simulink library "DAEMOT_Lib"  (R2019b)
settings: Solver=ode45  StartTime=0.0  StopTime=10.0  FixedStep=0.1  RelTol=1e-3
undefined symbols (not defined in the file or in its folder): Controller, CP, Ctrl, Ctrl_Fcn, Elec1, f, F2, Fluid, lag1, Mission, Moody, PropellerProp, rev_comms_sink
libraries: $bdroot x200, instrumentlib x21, simulink x5, dspsigops x2
(part 9 of 13)

== system DAEMOT_Lib/Legacy Components/LabVIEW_UDP_old ==
  " " : Inport
  Bus Creator : BusCreator  Inputs=46
  Bus Selector : BusSelector  OutputSignals=Temp1_Enabled,Temp2_Enabled,Temp3_Enabled,Temp4_Enabled,Temp5_Enabled,Temp6_Enabled,Temp7_Enabled,Temp8_Enabled,Temp9_Enabled,Temp10_Enabled,Temp11_Enabled,Temp12_Enabled,Temp13_Enabled,Temp14_Enabled,Temp15_Enabled,Temp16_Enabled,FlowMeter1_Enabled,FlowMeter2_Enabled,FlowMeter3_Enabled,FlowMeter4_Enabled,FlowMeter5_Enabled,FlowMeter6_Enabled,FlowMeter7_Enabled,FlowMeter8_Enabled,Pump1,Pump2,Pump3,Pump4,Pump5,Pump6,Pump7,Pump8,Pump1_Enabled,Pump2_Enabled,Pump3_Enabled,Pump4_Enabled,Pump5_Enabled,Pump6_Enabled,Pump7_Enabled,Pump8_Enabled,Heater1,Heater2,Heater3,Heater4,Heater1_Enabled,Heater2_Enabled,Heater3_Enabled,Heater4_Enabled,Heater1_CM_Enabled,Heater2_CM_Enabled,Heater3_CM_Enabled,Heater4_CM_Enabled,Pressure1_Enabled,Pressure2_Enabled,Pressure3_Enabled,Pressure4_Enabled,Pressure5_Enabled,Pressure6_Enabled,Pressure7_Enabled,Chiller2,Chiller2_Enabled,Valve1_Enabled,Valve2_Enabled,Valve3_Enabled,Valve4_Enabled,Valve5_Enabled,Valve6_Enabled,Valve7_Enabled,Valve8_Enabled,Chiller1,Chiller1_Enabled  OutputAsBus=on
  Bus to Vector : BusToVector
  Demux : Demux  Outputs=46
  UDP Receive : instrumentlib/UDP Receive  Host=localhost  Port=61556  LocalPort=61557  EnablePortSharing=off  GetLatestData=off  DataSize=[48 1]  DataType=double  ASCIIFormatting=%f,  Terminator=LF  ByteOrder=BigEndian  EnableBlockingMode=on  Timeout=10  SampleTime=0.1  LocalAddress=0.0.0.0
      settings: SourceProductName=Instrument Control Toolbox
  UDP Send : instrumentlib/UDP Send  Host=localhost  Port=61556  LocalPort=61557  EnablePortSharing=off  ByteOrder=BigEndian  OutputDatagramPacketSize=512  EnableBlockingMode=on  LocalAddress=0.0.0.0
      settings: SourceProductName=Instrument Control Toolbox
  Zero-Order Hold : ZeroOrderHold  Commented=through  SampleTime=0.1
  Out : Outport  VectorParamsAs1DForOutWhenUnconnected=off
  wires:
  UDP Receive/1 -> Demux/1
  Demux/1 -> Bus Creator/1  "Temp1"
  Demux/2 -> Bus Creator/2  "Temp2"
  Bus Creator/1 -> Out/1
  Demux/3 -> Bus Creator/3  "Temp3"
  Demux/4 -> Bus Creator/4  "Temp4"
  Demux/5 -> Bus Creator/5  "Temp5"
  Demux/6 -> Bus Creator/6  "Temp6"
  Demux/7 -> Bus Creator/7  "Temp7"
  Demux/8 -> Bus Creator/8  "Temp8"
  Demux/9 -> Bus Creator/9  "Temp9"
  Demux/10 -> Bus Creator/10  "Temp10"
  Demux/11 -> Bus Creator/11  "Temp11"
  Demux/12 -> Bus Creator/12  "Temp12"
  Demux/13 -> Bus Creator/13  "Temp13"
  Demux/14 -> Bus Creator/14  "Temp14"
  Demux/15 -> Bus Creator/15  "Temp15"
  Demux/16 -> Bus Creator/16  "Temp16"
  Demux/17 -> Bus Creator/17  "FlowMeter1"
  Demux/18 -> Bus Creator/18  "FlowMeter2"
  Demux/19 -> Bus Creator/19  "FlowMeter3"
  Demux/20 -> Bus Creator/20  "FlowMeter4"
  Demux/21 -> Bus Creator/21  "FlowMeter5"
  Demux/22 -> Bus Creator/22  "FlowMeter6"
  Demux/23 -> Bus Creator/23  "FlowMeter7"
  Demux/24 -> Bus Creator/24  "FlowMeter8"
  Demux/25 -> Bus Creator/25  "Pump1"
  Demux/26 -> Bus Creator/26  "Pump2"
  Demux/27 -> Bus Creator/27  "Pump3"
  Demux/28 -> Bus Creator/28  "Pump4"
  Demux/29 -> Bus Creator/29  "Pump5"
  Demux/30 -> Bus Creator/30  "Pump6"
  Demux/31 -> Bus Creator/31  "Pump7"
  Demux/32 -> Bus Creator/32  "Pump8"
  Demux/33 -> Bus Creator/33  "Heater1"
  Demux/34 -> Bus Creator/34  "Heater2"
  Demux/35 -> Bus Creator/35  "Heater3"
  Demux/36 -> Bus Creator/36  "Heater4"
  Demux/37 -> Bus Creator/37  "Pressure1"
  Demux/38 -> Bus Creator/38  "Pressure2"
  " "/1 -> Bus Selector/1
  Zero-Order Hold/1 -> UDP Send/1
  Bus Selector/1 -> Bus to Vector/1
  Bus to Vector/1 -> Zero-Order Hold/1
  Demux/39 -> Bus Creator/39  "Pressure3"
  Demux/40 -> Bus Creator/40  "Pressure4"
  Demux/41 -> Bus Creator/41  "Pressure5"
  Demux/42 -> Bus Creator/42  "Pressure6"
  Demux/43 -> Bus Creator/43  "Pressure7"
  Demux/44 -> Bus Creator/44  "Chiller1_flow"
  Demux/45 -> Bus Creator/45  "Chiller1_temp"
  Demux/46 -> Bus Creator/46  "RunTime"

== system DAEMOT_Lib/Legacy Components/Load ==
  In1 : Inport
  In2 : Inport  Port=2
  Bus Selector : BusSelector  OutputSignals=V,I
  Constant : Constant  Value=0
  Constant1 : Constant  Value=0
  Data_Sink1 : $bdroot/Support Functions/Data_Sink
  Divide : Product  Inputs=/
  Gain : Gain  Gain=1000
  P : Constant  Value=P_max
  Product : Product
  Product1 : Product
  Sink1 : $bdroot/Support Functions/Sink
  Switch : Switch  Criteria=u2 > Threshold
  Switch1 : Switch  Criteria=u2 > Threshold
  Terminator3 : Terminator
  b1 : BusCreator  Inputs=1
  wires:
  Bus Selector/1 -> Switch1/2, Divide/1, Switch/2  "<V>"
  Bus Selector/2 -> Terminator3/1  "<I>"
  Product1/1 -> Gain/1  "I"
  In1/1 -> Bus Selector/1
  P/1 -> Product/1
  In2/1 -> Product/2
  Switch/1 -> Product1/1
  Divide/1 -> Switch/1
  Constant/1 -> Switch/3
  b1/1 -> Data_Sink1/1
  Switch1/1 -> b1/1, Product1/2  "Power"
  Constant1/1 -> Switch1/3
  Product/1 -> Switch1/1  "Power"
  Gain/1 -> Sink1/1

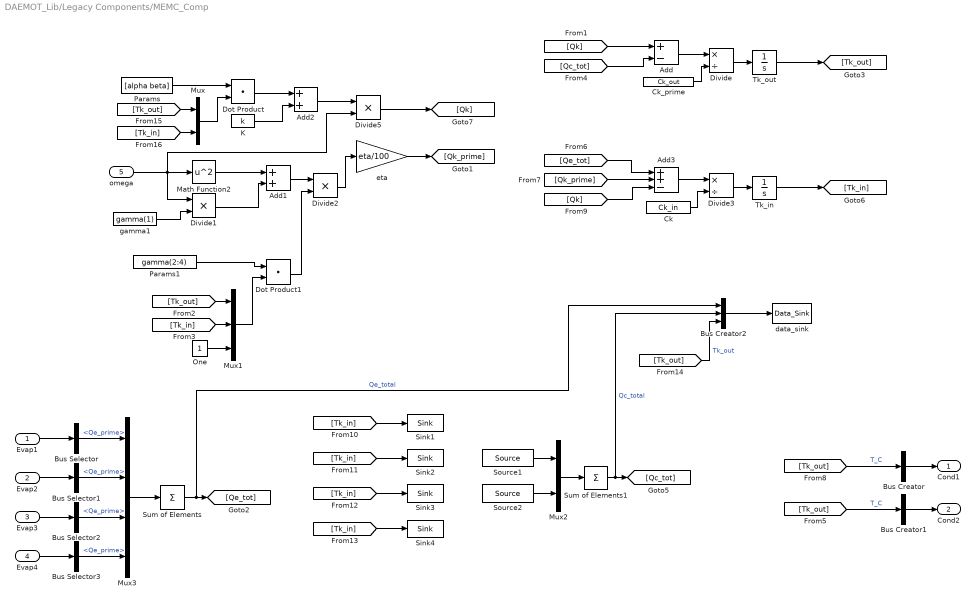
== system DAEMOT_Lib/Legacy Components/MEMC_Comp ==
  Evap1 : Inport
  Evap2 : Inport  Port=2
  Evap3 : Inport  Port=3
  Evap4 : Inport  Port=4
  omega : Inport  Port=5
  Add : Sum  Inputs=+-
  Add1 : Sum
  Add2 : Sum
  Add3 : Sum  Inputs=++-
  Bus Creator : BusCreator  Inputs=1
  Bus Creator1 : BusCreator  Inputs=1
  Bus Creator2 : BusCreator  Inputs=3
  Bus Selector{,1..3} (4 alike) : BusSelector  OutputSignals=Qe_prime
  Ck : Constant  Value=Ck_in
  Ck_prime : Constant  Value=Ck_out
  Divide : Product  Inputs=*/
  Divide1 : Product  Inputs=**
  Divide2 : Product  Inputs=**
  Divide3 : Product  Inputs=*/
  Divide5 : Product  Inputs=**
  Dot Product : DotProduct  InputSameDT=on  OutDataTypeStr=Inherit: Inherit via internal rule
  Dot Product1 : DotProduct  InputSameDT=on  OutDataTypeStr=Inherit: Inherit via internal rule
  K : Constant  Value=k
  Math Function2 : Math  Operator=square  SaturateOnIntegerOverflow=on
  Mux : Mux  Inputs=2
  Mux1 : Mux  Inputs=3
  Mux2 : Mux  Inputs=2
  Mux3 : Mux
  One : Constant
  Params : Constant  Value=[alpha beta]
  Params1 : Constant  Value=gamma(2:4)
  Sink{1..4} (4 alike) : $bdroot/Support Functions/Sink
  Source1 : $bdroot/Support Functions/Source
  Source2 : $bdroot/Support Functions/Source
  Sum of Elements : Sum  Inputs=+
  Sum of Elements1 : Sum  Inputs=+
  Tk_in : Integrator  InitialCondition=Tk_in_init
  Tk_out : Integrator  InitialCondition=Tk_out_init
  data_sink : $bdroot/Support Functions/Data_Sink
  eta : Gain  Gain=eta/100
  gamma1 : Constant  Value=gamma(1)
  Cond1 : Outport  VectorParamsAs1DForOutWhenUnconnected=off
  Cond2 : Outport  Port=2  VectorParamsAs1DForOutWhenUnconnected=off
  wires:
  [Tk_in] -> Sink4/1
  [Tk_in] -> Sink3/1
  [Tk_in] -> Sink2/1
  [Tk_in] -> Sink1/1
  [Qk] -> Add3/3
  Tk_in/1 -> [Tk_in]
  Add3/1 -> Divide3/1
  [Qk_prime] -> Add3/2
  [Qe_tot] -> Add3/1
  Divide3/1 -> Tk_in/1
  Ck/1 -> Divide3/2
  Sum of Elements1/1 -> Bus Creator2/2, [Qc_tot]  "Qc_total"
  Mux2/1 -> Sum of Elements1/1
  Source2/1 -> Mux2/2
  Source1/1 -> Mux2/1
  [Tk_out] -> Bus Creator1/1  "T_C"
  Bus Creator1/1 -> Cond2/1
  [Tk_out] -> Bus Creator/1  "T_C"
  Bus Creator/1 -> Cond1/1
  Tk_out/1 -> [Tk_out]
  Add/1 -> Divide/1
  [Qc_tot] -> Add/2
  [Qk] -> Add/1
  Divide/1 -> Tk_out/1
  Ck_prime/1 -> Divide/2
  Mux/1 -> Dot Product/2
  Params/1 -> Dot Product/1
  [Tk_in] -> Mux/2
  [Tk_out] -> Mux/1
  Divide5/1 -> [Qk]
  eta/1 -> [Qk_prime]
  Divide2/1 -> eta/1
  omega/1 -> Math Function2/1, Divide1/1, Divide5/2
  Add1/1 -> Divide2/1
  Math Function2/1 -> Add1/1
  Divide1/1 -> Add1/2
  gamma1/1 -> Divide1/2
  Mux1/1 -> Dot Product1/2
  Params1/1 -> Dot Product1/1
  [Tk_in] -> Mux1/2
  [Tk_out] -> Mux1/1
  Dot Product1/1 -> Divide2/2
  Dot Product/1 -> Add2/1
  K/1 -> Add2/2
  Add2/1 -> Divide5/1
  One/1 -> Mux1/3
  Sum of Elements/1 -> Bus Creator2/1, [Qe_tot]  "Qe_total"
  Mux3/1 -> Sum of Elements/1
  Bus Selector/1 -> Mux3/1  "<Qe_prime>"
  Bus Selector3/1 -> Mux3/4  "<Qe_prime>"
  Bus Selector1/1 -> Mux3/2  "<Qe_prime>"
  Bus Selector2/1 -> Mux3/3  "<Qe_prime>"
  Evap2/1 -> Bus Selector1/1
  Evap3/1 -> Bus Selector2/1
  Evap4/1 -> Bus Selector3/1
  Evap1/1 -> Bus Selector/1
  Bus Creator2/1 -> data_sink/1
  [Tk_out] -> Bus Creator2/3  "Tk_out"

== system DAEMOT_Lib/Legacy Components/MEMC_Valves ==
  Cond2 : Inport
  Cond1 : Inport  Port=2
  Add : Sum  Inputs=+-
  Bus Creator{,1..4} (5 alike) : BusCreator  Inputs=1
  Bus Selector1 : BusSelector  OutputSignals=Qc_prime
  Bus Selector2 : BusSelector  OutputSignals=Qc_prime
  Cv : Constant  Value=Cv
  Divide : Product  Inputs=*/
  Mux1 : Mux
  Mux2 : Mux  Inputs=2
  Sink1 : $bdroot/Support Functions/Sink
  Sink2 : $bdroot/Support Functions/Sink
  Source{1..4} (4 alike) : $bdroot/Support Functions/Source
  Sum of Elements1 : Sum  Inputs=+
  Sum of Elements4 : Sum  Inputs=+
  Tv : Integrator  InitialCondition=T_init
  data_sink : $bdroot/Support Functions/Data_Sink
  Evap4 : Outport  VectorParamsAs1DForOutWhenUnconnected=off
  Evap3 : Outport  Port=2  VectorParamsAs1DForOutWhenUnconnected=off
  Evap2 : Outport  Port=3  VectorParamsAs1DForOutWhenUnconnected=off
  Evap1 : Outport  Port=4  VectorParamsAs1DForOutWhenUnconnected=off
  wires:
  Tv/1 -> Bus Creator4/1, [Tv]  "Temp_C"
  Add/1 -> Divide/1
  [Qe_tot] -> Add/2
  [Qc_prime_tot] -> Add/1
  Divide/1 -> Tv/1
  Cv/1 -> Divide/2
  [Tv] -> Bus Creator/1, Bus Creator1/1, Bus Creator2/1, Bus Creator3/1  "T_C"
  Mux1/1 -> Sum of Elements4/1
  Sum of Elements4/1 -> [Qe_tot]
  Source4/1 -> Mux1/4
  Source3/1 -> Mux1/3
  Source1/1 -> Mux1/1
  Source2/1 -> Mux1/2
  Sum of Elements1/1 -> [Qc_prime_tot]
  Mux2/1 -> Sum of Elements1/1
  Bus Selector2/1 -> Mux2/2  "<Qc_prime>"
  Bus Selector1/1 -> Mux2/1  "<Qc_prime>"
  Cond2/1 -> Bus Selector1/1
  [Tv] -> Sink2/1, Sink1/1
  Bus Creator/1 -> Evap4/1
  Cond1/1 -> Bus Selector2/1
  Bus Creator1/1 -> Evap3/1
  Bus Creator2/1 -> Evap2/1
  Bus Creator3/1 -> Evap1/1
  Bus Creator4/1 -> data_sink/1

== system DAEMOT_Lib/Legacy Components/Pipe_M_to_M ==
  In1 : Inport
  In2 : Inport  Port=2
  Add1 : Sum
  Add5 : Sum
  Bus Creator2 : BusCreator  Inputs=3
  Constant : Constant  Value=4/(pi*D)
  Constant1 : Constant  Value=e/D
  Display : Display
  Display1 : Display
  Display2 : Display
  Divide5 : Product  Inputs=**/
  From1 : From  Commented=on  GotoTag=T_out
      settings: CloseFcn=tagdialog Close
  Gain1 : Gain  Gain=1/Fluid.Bulk_Mod
  Gain2 : Gain  Gain=0.5
  Gain3 : Gain  Gain=0.5
  Integrate1 : Integrator  InitialCondition=P_init
  Memory1 : Memory  Commented=on  InitialCondition=[Tout_init]
  Pipe_M_to_M : MATLAB Function  TreatAsAtomicUnit=on
  Props : Subsystem
  Sink1 : $bdroot/Support Functions/Sink
  Source1 : $bdroot/Support Functions/Source
  Terminator : Terminator
  Terminator1 : Terminator
  Terminator2 : Terminator
  b1 : BusCreator  Inputs=3
  data_sink1 : $bdroot/Support Functions/Data_Sink
  gb1 : BusSelector  OutputSignals=mdot_kgps,T_C,P_kPa
  n-D Lookup Table5 : Lookup_n-D  BreakpointsForDimension1=Moody.Re_vec  BreakpointsForDimension2=Moody.eD_vec  BreakpointsForDimension3=[5, 7]  Table=Moody.f  ExtrapMethod=Clip  UseLastTableValue=on  RndMeth=Simplest  InputSameDT=on
  n-D Lookup Table9 : Lookup_n-D  BreakpointsForDimension1=Fluid.P  BreakpointsForDimension2=Fluid.T  BreakpointsForDimension3=[5, 7]  Table=Fluid.Mu_pt  RndMeth=Simplest  InputSameDT=on
  Out1 : Outport  VectorParamsAs1DForOutWhenUnconnected=off
  wires:
  b1/1 -> Out1/1
  [Mdot_out] -> b1/1  "mdot_kgps"
  gb1/2 -> [T_in]  "<T_C>"
  [T_out] -> b1/2  "T_C"
  gb1/1 -> [Mdot_in]  "<mdot_kgps>"
  In1/1 -> gb1/1
  [P_out] -> b1/3  "P_kPa"
  gb1/3 -> Terminator/1  "<P_kPa>"
  [P_in] -> Sink1/1
  Source1/1 -> [Mdot_out]
  In2/1 -> [T_amb]
  Bus Creator2/1 -> data_sink1/1
  [T_out] -> Bus Creator2/1  "T_out"
  [P_in] -> Bus Creator2/2  "P_in"
  [T_amb] -> Terminator1/1
  [T_in] -> [T_out]
  [Mdot_in] -> Add5/1, Pipe_M_to_M/2(Mdot_in)
  [Mdot_out] -> Add5/2, Pipe_M_to_M/3(Mdot_out)
  [T_in] -> Add1/2, Add1/1
  From1/1 -> Memory1/1
  Add1/1 -> Gain2/1
  Gain2/1 -> n-D Lookup Table9/2, Props/2(T)
  [P] -> Props/1(P), n-D Lookup Table9/1
  Add5/1 -> Gain3/1
  Constant/1 -> Divide5/1
  Gain3/1 -> Divide5/2
  Divide5/1 -> Display/1, n-D Lookup Table5/1  "Re"
  Constant1/1 -> Display2/1, n-D Lookup Table5/2
  n-D Lookup Table5/1 -> Pipe_M_to_M/6(f), Display1/1
  Props/1(Rho) -> Gain1/1, Pipe_M_to_M/4(Rho)
  Integrate1/1 -> [P], Pipe_M_to_M/1(x)
  Pipe_M_to_M/1(x_dot) -> Integrate1/1
  [P_out] -> Bus Creator2/3  "P_out"
  Pipe_M_to_M/2(P_in) -> [P_in]
  Pipe_M_to_M/3(P_out) -> [P_out]
  n-D Lookup Table9/1 -> Divide5/3  "mu"
  Gain1/1 -> Pipe_M_to_M/5(dRho_dP)
  Props/2(dRho_dP) -> Terminator2/1

== system DAEMOT_Lib/Legacy Components/Pipe_M_to_P ==
  In1 : Inport
  In2 : Inport  Port=2
  Add1 : Sum
  Bus Creator2 : BusCreator  Inputs=3
  Constant : Constant  Value=4/(pi*D)
  Constant1 : Constant  Value=e/D
  Display : Display
  Display1 : Display
  Display2 : Display
  Divide5 : Product  Inputs=**/
  From1 : From  Commented=on  GotoTag=T_out
      settings: CloseFcn=tagdialog Close
  Gain1 : Gain  Gain=1/Fluid.Bulk_Mod
  Gain2 : Gain  Gain=0.5
  Integrate : Integrator  InitialCondition=P_init
  Memory1 : Memory  Commented=on  InitialCondition=[Tout_init]
  Pipe_P_to_M : MATLAB Function  TreatAsAtomicUnit=on
  Sink1 : $bdroot/Support Functions/Sink
  Source1 : $bdroot/Support Functions/Source
  Terminator1 : Terminator
  Terminator2 : Terminator
  b2 : BusCreator  Inputs=3
  data_sink1 : $bdroot/Support Functions/Data_Sink
  gb2 : BusSelector  OutputSignals=mdot_kgps,T_C,P_kPa
  n-D Lookup Table2 : Lookup_n-D  BreakpointsForDimension1=Fluid.P  BreakpointsForDimension2=Fluid.T  BreakpointsForDimension3=[5, 7]  Table=Fluid.Rho_pt  ExtrapMethod=Clip  UseLastTableValue=on  RndMeth=Simplest  InputSameDT=on
  n-D Lookup Table5 : Lookup_n-D  BreakpointsForDimension1=Moody.Re_vec  BreakpointsForDimension2=Moody.eD_vec  BreakpointsForDimension3=[5, 7]  Table=Moody.f  ExtrapMethod=Clip  UseLastTableValue=on  RndMeth=Simplest  InputSameDT=on
  n-D Lookup Table9 : Lookup_n-D  BreakpointsForDimension1=Fluid.P  BreakpointsForDimension2=Fluid.T  BreakpointsForDimension3=[5, 7]  Table=Fluid.Mu_pt  RndMeth=Simplest  InputSameDT=on
  Out1 : Outport  VectorParamsAs1DForOutWhenUnconnected=off
  wires:
  Bus Creator2/1 -> data_sink1/1
  [T_out] -> Bus Creator2/1  "T_out"
  [T_amb] -> Terminator1/1
  [T_in] -> [T_out]
  From1/1 -> Memory1/1
  Add1/1 -> Gain2/1
  Gain2/1 -> n-D Lookup Table2/2, n-D Lookup Table9/2
  [P_in] -> n-D Lookup Table2/1, n-D Lookup Table9/1
  Constant/1 -> Divide5/1
  Divide5/1 -> Display/1, n-D Lookup Table5/1  "Re"
  Constant1/1 -> Display2/1, n-D Lookup Table5/2
  n-D Lookup Table5/1 -> Pipe_P_to_M/6(f), Display1/1
  n-D Lookup Table2/1 -> Pipe_P_to_M/4(Rho), Gain1/1
  [T_in] -> Add1/2, Add1/1
  n-D Lookup Table9/1 -> Divide5/3  "mu"
  [Mdot] -> Bus Creator2/2  "Mdot"
  Pipe_P_to_M/2(Mdot) -> [Mdot]
  [P_in] -> Bus Creator2/3  "P_out"
  [Mdot_up] -> Divide5/2
  Pipe_P_to_M/1(x_dot) -> Integrate/1
  Integrate/1 -> Pipe_P_to_M/1(x), [P_in]
  b2/1 -> Out1/1
  [Mdot] -> b2/1  "mdot_kgps"
  gb2/2 -> [T_in]  "<T_C>"
  [T_out] -> b2/2  "T_C"
  gb2/1 -> [Mdot_up]  "<mdot_kgps>"
  In1/1 -> gb2/1
  [P_out] -> b2/3  "P_kPa"
  gb2/3 -> Terminator2/1  "<P_kPa>"
  [P_in] -> Sink1/1
  Source1/1 -> [P_out]
  In2/1 -> [T_amb]
  [P_out] -> Pipe_P_to_M/2(P_out)
  [Mdot_up] -> Pipe_P_to_M/3(Mdot_up)
  Gain1/1 -> Pipe_P_to_M/5(dRho_dP)

== system DAEMOT_Lib/Legacy Components/Pipe_P_to_M1 ==
  In1 : Inport
  Bus Creator2 : BusCreator  Inputs=3
  Constant2 : Constant  Value=Fluid.Bulk_Mod
  Demux : Demux  Outputs=2
  Integrate : Integrator  InitialCondition=[T_init P_init]
  Mdot : MATLAB Function  TreatAsAtomicUnit=on
  Pipe_P_to_M : MATLAB Function  TreatAsAtomicUnit=on
  Sink1 : $bdroot/Support Functions/Sink
  Source1 : $bdroot/Support Functions/Source
  Terminator3 : Terminator
  b2 : BusCreator  Inputs=3
  data_sink1 : $bdroot/Support Functions/Data_Sink
  gb2 : BusSelector  OutputSignals=mdot_kgps,T_C,P_kPa
  n-D Lookup Table2 : Lookup_n-D  BreakpointsForDimension1=Fluid.P  BreakpointsForDimension2=Fluid.T  BreakpointsForDimension3=[5, 7]  Table=Fluid.Rho_pt  ExtrapMethod=Clip  UseLastTableValue=on  RndMeth=Simplest  InputSameDT=on
  Out1 : Outport  VectorParamsAs1DForOutWhenUnconnected=off
  wires:
  Bus Creator2/1 -> data_sink1/1
  [T_out] -> Bus Creator2/1  "T_out"
  [T_out] -> n-D Lookup Table2/2
  [P_out] -> n-D Lookup Table2/1
  n-D Lookup Table2/1 -> Pipe_P_to_M/5(Rho), Mdot/3(Rho)
  [Mdot] -> Bus Creator2/2  "Mdot"
  [P_out] -> Bus Creator2/3  "P_out"
  Pipe_P_to_M/1(x_dot) -> Integrate/1
  Integrate/1 -> Pipe_P_to_M/1(x), Demux/1
  b2/1 -> Out1/1
  [Mdot_down] -> b2/1  "mdot_kgps"
  gb2/2 -> [T_in]  "<T_C>"
  [T_out] -> b2/2  "T_C"
  gb2/1 -> Terminator3/1  "<mdot_kgps>"
  In1/1 -> gb2/1
  [P_out] -> b2/3  "P_kPa"
  gb2/3 -> [P_in]  "<P_kPa>"
  [Mdot] -> Sink1/1
  Source1/1 -> [Mdot_down]
  [Mdot_down] -> Pipe_P_to_M/3(Mdot_down)
  Constant2/1 -> Pipe_P_to_M/6(E_fluid)
  [T_in] -> Pipe_P_to_M/2(T_in)
  [P_in] -> Mdot/1(P_in)
  [P_out] -> Mdot/2(P_out)
  Mdot/1(Mdot) -> Pipe_P_to_M/4(Mdot), [Mdot]
  Demux/2 -> [P_out]
  Demux/1 -> [T_out]

== system DAEMOT_Lib/Legacy Components/Pipe_P_to_M_Wall ==
  In1 : Inport
  In2 : Inport  Port=2
  Bus Creator2 : BusCreator  Inputs=4
  Constant2 : Constant  Value=Fluid.Bulk_Mod
  Demux : Demux  Outputs=2
  Integrate : Integrator  InitialCondition=[T_init P_init]
  Mdot : MATLAB Function  TreatAsAtomicUnit=on
  Pipe_P_to_M : MATLAB Function  TreatAsAtomicUnit=on
  Sink1 : $bdroot/Support Functions/Sink
  Sink2 : $bdroot/Support Functions/Sink
  Source1 : $bdroot/Support Functions/Source
  Terminator3 : Terminator
  b2 : BusCreator  Inputs=3
  bus : BusSelector  OutputSignals=T_wall
  data_sink1 : $bdroot/Support Functions/Data_Sink
  gb2 : BusSelector  OutputSignals=mdot_kgps,T_C,P_kPa
  n-D Lookup Table1 : Lookup_n-D  BreakpointsForDimension1=Fluid.P  BreakpointsForDimension2=Fluid.T  BreakpointsForDimension3=[5, 7]  Table=Fluid.C_pt  ExtrapMethod=Clip  UseLastTableValue=on  RndMeth=Simplest  InputSameDT=on
  n-D Lookup Table2 : Lookup_n-D  BreakpointsForDimension1=Fluid.P  BreakpointsForDimension2=Fluid.T  BreakpointsForDimension3=[5, 7]  Table=Fluid.Rho_pt  ExtrapMethod=Clip  UseLastTableValue=on  RndMeth=Simplest  InputSameDT=on
  n-D Lookup Table8 : Lookup_n-D  BreakpointsForDimension1=Fluid.P  BreakpointsForDimension2=Fluid.T  BreakpointsForDimension3=[5, 7]  Table=Fluid.K_pt  ExtrapMethod=Clip  UseLastTableValue=on  RndMeth=Simplest  InputSameDT=on
  n-D Lookup Table9 : Lookup_n-D  BreakpointsForDimension1=Fluid.P  BreakpointsForDimension2=Fluid.T  BreakpointsForDimension3=[5, 7]  Table=Fluid.Mu_pt  ExtrapMethod=Clip  UseLastTableValue=on  RndMeth=Simplest  InputSameDT=on
  Out1 : Outport  VectorParamsAs1DForOutWhenUnconnected=off
  wires:
  Bus Creator2/1 -> data_sink1/1
  [T_out] -> Bus Creator2/1  "T_out"
  In2/1 -> bus/1
  [T_out] -> n-D Lookup Table1/2, n-D Lookup Table8/2, n-D Lookup Table9/2, n-D Lookup Table2/2
  n-D Lookup Table2/1 -> Pipe_P_to_M/9(Rho), Mdot/3(Rho)
  [Mdot] -> Bus Creator2/2  "Mdot"
  [P_out] -> Bus Creator2/3  "P_out"
  Pipe_P_to_M/1(x_dot) -> Integrate/1
  Integrate/1 -> Pipe_P_to_M/1(x), Demux/1
  b2/1 -> Out1/1
  [Mdot_down] -> b2/1  "mdot_kgps"
  gb2/2 -> [T_in]  "<T_C>"
  [T_out] -> b2/2  "T_C"
  gb2/1 -> Terminator3/1  "<mdot_kgps>"
  In1/1 -> gb2/1
  [P_out] -> b2/3  "P_kPa"
  gb2/3 -> [P_in]  "<P_kPa>"
  [Mdot] -> Sink1/1
  Source1/1 -> [Mdot_down]
  [Mdot_down] -> Pipe_P_to_M/3(Mdot_down)
  Constant2/1 -> Pipe_P_to_M/5(E_fluid)
  [T_in] -> Pipe_P_to_M/2(T_in)
  [P_in] -> Mdot/1(P_in)
  [P_out] -> Mdot/2(P_out)
  Mdot/1(Mdot) -> Pipe_P_to_M/4(Mdot), [Mdot]
  Demux/2 -> [P_out]
  Demux/1 -> [T_out]
  n-D Lookup Table9/1 -> Pipe_P_to_M/6(mu)
  n-D Lookup Table1/1 -> Pipe_P_to_M/8(Cp)
  n-D Lookup Table8/1 -> Pipe_P_to_M/7(k)
  [P_out] -> n-D Lookup Table2/1, n-D Lookup Table1/1, n-D Lookup Table9/1, n-D Lookup Table8/1
  Pipe_P_to_M/2(Q_kW) -> [Q_fluid]
  [Q_fluid] -> Bus Creator2/4  "Q"
  [Q_fluid] -> Sink2/1
  bus/1 -> Pipe_P_to_M/10(T_wall)  "<T_wall>"

== system DAEMOT_Lib/Legacy Components/Pipe_P_to_M_with_Heat_Load ==
  In1 : Inport
  Q : Inport  Port=2
  Bus Creator2 : BusCreator  Inputs=4
  Bus Selector : BusSelector  OutputSignals=Q_kW,Temp
  Constant2 : Constant  Value=Fluid.Bulk_Mod
  Demux : Demux  Outputs=2
  Integrate : Integrator  InitialCondition=[T_init P_init]
  Mdot : MATLAB Function  TreatAsAtomicUnit=on
  Pipe_P_to_M : MATLAB Function  TreatAsAtomicUnit=on
  Sink1 : $bdroot/Support Functions/Sink
  Sink2 : $bdroot/Support Functions/Sink
  Source1 : $bdroot/Support Functions/Source
  Terminator : Terminator
  Terminator3 : Terminator
  b2 : BusCreator  Inputs=3
  data_sink1 : $bdroot/Support Functions/Data_Sink
  gb2 : BusSelector  OutputSignals=mdot_kgps,T_C,P_kPa
  n-D Lookup Table1 : Lookup_n-D  BreakpointsForDimension1=Fluid.P  BreakpointsForDimension2=Fluid.T  BreakpointsForDimension3=[5, 7]  Table=Fluid.C_pt  ExtrapMethod=Clip  UseLastTableValue=on  RndMeth=Simplest  InputSameDT=on
  n-D Lookup Table2 : Lookup_n-D  BreakpointsForDimension1=Fluid.P  BreakpointsForDimension2=Fluid.T  BreakpointsForDimension3=[5, 7]  Table=Fluid.Rho_pt  ExtrapMethod=Clip  UseLastTableValue=on  RndMeth=Simplest  InputSameDT=on
  Out1 : Outport  VectorParamsAs1DForOutWhenUnconnected=off
  wires:
  [Q_Load] -> Pipe_P_to_M/7(Q_load)
  [T_out] -> Sink2/1
  Bus Selector/2 -> Terminator/1  "<Temp>"
  Q/1 -> Bus Selector/1
  Bus Selector/1 -> [Q_Load]  "<Q_kW>"
  Bus Creator2/1 -> data_sink1/1
  [T_out] -> Bus Creator2/1  "T_out"
  [T_out] -> n-D Lookup Table1/2, n-D Lookup Table2/2
  [P_out] -> n-D Lookup Table1/1, n-D Lookup Table2/1
  n-D Lookup Table2/1 -> Pipe_P_to_M/5(Rho), Mdot/3(Rho)
  [Mdot] -> Bus Creator2/2  "Mdot"
  [P_out] -> Bus Creator2/3  "P_out"
  Pipe_P_to_M/1(x_dot) -> Integrate/1
  Integrate/1 -> Pipe_P_to_M/1(x), Demux/1
  b2/1 -> Out1/1
  [Mdot_down] -> b2/1  "mdot_kgps"
  gb2/2 -> [T_in]  "<T_C>"
  [T_out] -> b2/2  "T_C"
  gb2/1 -> Terminator3/1  "<mdot_kgps>"
  In1/1 -> gb2/1
  [P_out] -> b2/3  "P_kPa"
  gb2/3 -> [P_in]  "<P_kPa>"
  [Mdot] -> Sink1/1
  Source1/1 -> [Mdot_down]
  [Mdot_down] -> Pipe_P_to_M/3(Mdot_down)
  Constant2/1 -> Pipe_P_to_M/6(E_fluid)
  [T_in] -> Pipe_P_to_M/2(T_in)
  [P_in] -> Mdot/1(P_in)
  [P_out] -> Mdot/2(P_out)
  Mdot/1(Mdot) -> Pipe_P_to_M/4(Mdot), [Mdot]
  Demux/2 -> [P_out]
  Demux/1 -> [T_out]
  [Q_Load] -> Bus Creator2/4  "Q_load"
  n-D Lookup Table1/1 -> Pipe_P_to_M/8(Cp)

== system DAEMOT_Lib/Legacy Components/Pipe_P_to_P1 ==
  In1 : Inport
  Bus Creator2 : BusCreator  Inputs=2
  Integrate1 : Integrator  InitialCondition=T_init
  Mdot : MATLAB Function  TreatAsAtomicUnit=on
  Pipe_P_to_M : MATLAB Function  TreatAsAtomicUnit=on
  Sink1 : $bdroot/Support Functions/Sink
  Source1 : $bdroot/Support Functions/Source
  Terminator2 : Terminator
  b1 : BusCreator  Inputs=3
  data_sink1 : $bdroot/Support Functions/Data_Sink
  gb1 : BusSelector  OutputSignals=mdot_kgps,T_C,P_kPa
  n-D Lookup Table1 : Lookup_n-D  BreakpointsForDimension1=Fluid.P  BreakpointsForDimension2=Fluid.T  BreakpointsForDimension3=[5, 7]  Table=Fluid.Rho_pt  ExtrapMethod=Clip  UseLastTableValue=on  RndMeth=Simplest  InputSameDT=on
  Out1 : Outport  VectorParamsAs1DForOutWhenUnconnected=off
  wires:
  b1/1 -> Out1/1
  [Mdot] -> b1/1  "mdot_kgps"
  gb1/2 -> [T_in]  "<T_C>"
  [T_out] -> b1/2  "T_C"
  gb1/1 -> Terminator2/1  "<mdot_kgps>"
  In1/1 -> gb1/1
  [P_out] -> b1/3  "P_kPa"
  gb1/3 -> [P_in]  "<P_kPa>"
  [Mdot] -> Sink1/1
  Source1/1 -> [P_out]
  Bus Creator2/1 -> data_sink1/1
  [T_out] -> Bus Creator2/1  "T_out"
  [Mdot] -> Bus Creator2/2  "Mdot"
  Pipe_P_to_M/1(x_dot) -> Integrate1/1
  Integrate1/1 -> Pipe_P_to_M/1(x), [T_out]
  [T_in] -> Pipe_P_to_M/2(T_in)
  [T_out] -> n-D Lookup Table1/2
  [P_out] -> n-D Lookup Table1/1
  n-D Lookup Table1/1 -> Mdot/3(Rho), Pipe_P_to_M/4(Rho)
  [P_in] -> Mdot/1(P_in)
  [P_out] -> Mdot/2(P_out)
  Mdot/1(Mdot) -> [Mdot], Pipe_P_to_M/3(Mdot)

== system DAEMOT_Lib/Legacy Components/Power Sink (Current) ==
  In1 : Inport
  In2 : Inport  Port=2
  Sink1 : Subsystem  LoadFcn=rev_comms_sink();  InitFcn=rev_comms_sink();  mask(Sink){}
      mask help: Used for sending data to the upstream component.
      settings: CopyFcn=rev_comms_sink();  NameChangeFcn=rev_comms_sink();
      mask Display: text(0.25,0.5,'Sink')
  Terminator : Terminator
  wires:
  In2/1 -> Sink1/1(In1)  "current"
  In1/1 -> Terminator/1

== system DAEMOT_Lib/Legacy Components/Power Source (Voltage) ==
  In1 : Inport
  In2 : Inport  Port=2
  Source1 : Subsystem  mask(Source){}
      mask help: Used for receiving data from the downstream component.
      mask init:
      | n_src = gcb;
      | n_src = str2num(n_src(end));
      | try
      |     rev_comms_source(n_src);
      | catch
      | 
      | end
      mask Display: text(0.25,0.5,'Source')
  Terminator : Terminator
  b1 : BusCreator  Inputs=2
  Out1 : Outport  VectorParamsAs1DForOutWhenUnconnected=off
  wires:
  b1/1 -> Out1/1
  In2/1 -> b1/2  "voltage"
  In1/1 -> b1/1  "current"
  Source1/1(Out1) -> Terminator/1

== system DAEMOT_Lib/Legacy Components/Pump ==
  In1 : Inport
  In2 : Inport  Port=2
  In3 : Inport  Port=3
  Bus Creator2 : BusCreator  Inputs=7
  Constant1 : Constant  Value=T_init
  Constant11 : Constant  Value=T_init
  Constant2 : Constant  Value=P_init
  Constant7 : Constant  Value=P_init
  Data_Sink1 : $bdroot/Support Functions/Data_Sink
  Demux : Demux  Outputs=2
  Integrate : Integrator  InitialCondition=[T_init P_init]
  Pump : MATLAB Function  TreatAsAtomicUnit=on
  Sink1 : $bdroot/Support Functions/Sink
  Sink2 : $bdroot/Support Functions/Sink
  Source1 : $bdroot/Support Functions/Source
  Terminator1 : Terminator
  Terminator2 : Terminator
  b1 : BusCreator  Inputs=3
  gb1 : BusSelector  OutputSignals=mdot_kgps,T_C,P_kPa
  gb2 : BusSelector  OutputSignals=V,I
  n-D Lookup Table1 : Lookup_n-D  BreakpointsForDimension1=Fluid.P  BreakpointsForDimension2=Fluid.T  BreakpointsForDimension3=[5, 7]  Table=Fluid.C_pt  ExtrapMethod=Clip  UseLastTableValue=on  RndMeth=Simplest  InputSameDT=on
  n-D Lookup Table2 : Lookup_n-D  BreakpointsForDimension1=Fluid.P  BreakpointsForDimension2=Fluid.T  BreakpointsForDimension3=[5, 7]  Table=Fluid.Rho_pt  ExtrapMethod=Clip  UseLastTableValue=on  RndMeth=Simplest  InputSameDT=on
  Out1 : Outport  VectorParamsAs1DForOutWhenUnconnected=off
  wires:
  b1/1 -> Out1/1
  [Mdot_down] -> b1/1  "mdot_kgps"
  gb1/2 -> [T_in]  "<T_C>"
  [T_out] -> b1/2  "T_C"
  gb1/1 -> Terminator1/1  "<mdot_kgps>"
  In1/1 -> gb1/1
  [P_out] -> b1/3  "P_kPa"
  gb1/3 -> [P_in]  "<P_kPa>"
  [Mdot] -> Sink1/1
  Source1/1 -> [Mdot_down]
  In3/1 -> [Omega]
  [Omega] -> Pump/6(Omega)
  Pump/3(I) -> [I]
  Bus Creator2/1 -> Data_Sink1/1
  [T_out] -> Bus Creator2/1  "T_out"
  [Mdot] -> Bus Creator2/2  "Mdot"
  [I] -> Bus Creator2/4  "Current"
  [P_in] -> Pump/2(P_in)
  [Mdot_down] -> Pump/5(Mdot_down)
  Integrate/1 -> Pump/1(x), Demux/1
  Pump/1(x_dot) -> Integrate/1
  [T_in] -> Pump/3(T_in)
  [P_out] -> Bus Creator2/3  "P_out"
  Pump/2(Mdot) -> [Mdot]
  Demux/2 -> [P_out]
  Demux/1 -> [T_out]
  gb2/1 -> [V_in]  "<V>"
  In2/1 -> gb2/1
  gb2/2 -> Terminator2/1  "<I>"
  [I] -> Sink2/1
  [Omega] -> Bus Creator2/5  "Speed"
  [Q] -> Bus Creator2/6  "Q"
  Pump/4(Q) -> [Q]
  [V_in] -> Pump/4(V_in)
  Pump/5(eta) -> [eta]
  [eta] -> Bus Creator2/7  "eta"
  Constant7/1 -> n-D Lookup Table2/1
  Constant11/1 -> n-D Lookup Table2/2
  n-D Lookup Table2/1 -> Pump/7(rho)
  Constant2/1 -> n-D Lookup Table1/1
  Constant1/1 -> n-D Lookup Table1/2
  n-D Lookup Table1/1 -> Pump/8(cp)

== system DAEMOT_Lib/Legacy Components/QLoad ==
  In1 : Inport
  In2 : Inport  Port=2
  Bus Selector : BusSelector  OutputSignals=V,I
  Constant : Constant  Value=0
  Constant1 : Constant  Value=0
  Data_Sink1 : $bdroot/Support Functions/Data_Sink
  Divide : Product  Inputs=/
  Divide1 : Product  Inputs=*/
  Fcn : Fcn  Expr=1-u
  Gain : Gain  Gain=1000
  P : Constant  Value=P_max
  Product : Product
  Product1 : Product
  Product2 : Product
  Sink1 : $bdroot/Support Functions/Sink
  Source1 : $bdroot/Support Functions/Source
  Switch : Switch  Criteria=u2 > Threshold
  Switch1 : Switch  Criteria=u2 > Threshold
  Terminator3 : Terminator
  b1 : BusCreator  Inputs=3
  b2 : BusCreator  Inputs=2
  eta : Fcn  Expr=a*u^2+b*u+c
  Out1 : Outport  VectorParamsAs1DForOutWhenUnconnected=off
  wires:
  Bus Selector/1 -> Divide/1, Switch/2, Switch1/2  "<V>"
  Bus Selector/2 -> Terminator3/1  "<I>"
  Product1/1 -> Gain/1  "I"
  In1/1 -> Bus Selector/1
  P/1 -> Product/1
  In2/1 -> Product/2
  Switch/1 -> Product1/1
  Divide/1 -> Switch/1
  Constant/1 -> Switch/3
  b1/1 -> Data_Sink1/1
  Switch1/1 -> b1/2, Divide1/1  "Power"
  b2/1 -> Out1/1
  [T] -> b2/1  "T"
  [Q] -> b2/2  "Q_kW"
  Source1/1 -> [T]
  [T] -> eta/1
  eta/1 -> b1/1, Fcn/1, Divide1/2  "eta"
  Divide1/1 -> Product1/2, Product2/1  "P_in"
  Product2/1 -> [Q]
  Fcn/1 -> Product2/2
  Constant1/1 -> Switch1/3
  Product/1 -> Switch1/1  "Power"
  [Q] -> b1/3  "Q_kW"
  Gain/1 -> Sink1/1

== system DAEMOT_Lib/Legacy Components/Solenoid_P_to_M ==
  In1 : Inport
  In2 : Inport  Port=2
  Bus Creator2 : BusCreator  Inputs=3
  Constant : Constant  Value=0
  Constant2 : Constant  Value=Fluid.Bulk_Mod
  Demux : Demux  Outputs=2
  Integrate : Integrator  InitialCondition=[T_init P_init]
  Mdot : MATLAB Function  TreatAsAtomicUnit=on
  Pipe_P_to_M : MATLAB Function  TreatAsAtomicUnit=on
  Sink1 : $bdroot/Support Functions/Sink
  Source1 : $bdroot/Support Functions/Source
  Switch : Switch  Criteria=u2 > Threshold  Threshold=0.5
  Terminator3 : Terminator
  b2 : BusCreator  Inputs=3
  data_sink1 : $bdroot/Support Functions/Data_Sink
  gb2 : BusSelector  OutputSignals=mdot_kgps,T_C,P_kPa
  n-D Lookup Table2 : Lookup_n-D  BreakpointsForDimension1=Fluid.P  BreakpointsForDimension2=Fluid.T  BreakpointsForDimension3=[5, 7]  Table=Fluid.Rho_pt  ExtrapMethod=Clip  UseLastTableValue=on  RndMeth=Simplest  InputSameDT=on
  Out1 : Outport  VectorParamsAs1DForOutWhenUnconnected=off
  wires:
  Bus Creator2/1 -> data_sink1/1
  [T_out] -> Bus Creator2/1  "T_out"
  [T_out] -> n-D Lookup Table2/2
  [P_out] -> n-D Lookup Table2/1
  n-D Lookup Table2/1 -> Pipe_P_to_M/5(Rho), Mdot/3(Rho)
  [Mdot] -> Bus Creator2/2  "Mdot"
  [P_out] -> Bus Creator2/3  "P_out"
  Pipe_P_to_M/1(x_dot) -> Integrate/1
  Integrate/1 -> Pipe_P_to_M/1(x), Demux/1
  b2/1 -> Out1/1
  [Mdot_down] -> b2/1  "mdot_kgps"
  gb2/2 -> [T_in]  "<T_C>"
  [T_out] -> b2/2  "T_C"
  gb2/1 -> Terminator3/1  "<mdot_kgps>"
  In1/1 -> gb2/1
  [P_out] -> b2/3  "P_kPa"
  gb2/3 -> [P_in]  "<P_kPa>"
  [Mdot] -> Sink1/1
  Source1/1 -> [Mdot_down]
  In2/1 -> [On_off]
  [Mdot_down] -> Pipe_P_to_M/3(Mdot_down)
  Constant2/1 -> Pipe_P_to_M/6(E_fluid)
  [T_in] -> Pipe_P_to_M/2(T_in)
  [P_in] -> Mdot/1(P_in)
  [P_out] -> Mdot/2(P_out)
  Demux/2 -> [P_out]
  Demux/1 -> [T_out]
  Switch/1 -> Pipe_P_to_M/4(Mdot), [Mdot]
  Mdot/1(Mdot) -> Switch/1
  Constant/1 -> Switch/3
  [On_off] -> Switch/2

== system DAEMOT_Lib/Legacy Components/Solenoid_P_to_P ==
  In1 : Inport
  In2 : Inport  Port=2
  Bus Creator2 : BusCreator  Inputs=2
  Constant : Constant  Value=0
  Integrate1 : Integrator  InitialCondition=T_init
  Mdot : MATLAB Function  TreatAsAtomicUnit=on
  Pipe_P_to_M : MATLAB Function  TreatAsAtomicUnit=on
  Sink1 : $bdroot/Support Functions/Sink
  Source1 : $bdroot/Support Functions/Source
  Switch : Switch  Criteria=u2 > Threshold  Threshold=0.5
  Terminator2 : Terminator
  b1 : BusCreator  Inputs=3
  data_sink1 : $bdroot/Support Functions/Data_Sink
  gb1 : BusSelector  OutputSignals=mdot_kgps,T_C,P_kPa
  n-D Lookup Table1 : Lookup_n-D  BreakpointsForDimension1=Fluid.P  BreakpointsForDimension2=Fluid.T  BreakpointsForDimension3=[5, 7]  Table=Fluid.Rho_pt  ExtrapMethod=Clip  UseLastTableValue=on  RndMeth=Simplest  InputSameDT=on
  Out1 : Outport  VectorParamsAs1DForOutWhenUnconnected=off
  wires:
  b1/1 -> Out1/1
  [Mdot] -> b1/1  "mdot_kgps"
  gb1/2 -> [T_in]  "<T_C>"
  [T_out] -> b1/2  "T_C"
  gb1/1 -> Terminator2/1  "<mdot_kgps>"
  In1/1 -> gb1/1
  [P_out] -> b1/3  "P_kPa"
  gb1/3 -> [P_in]  "<P_kPa>"
  [Mdot] -> Sink1/1
  Source1/1 -> [P_out]
  In2/1 -> [On_off]
  Bus Creator2/1 -> data_sink1/1
  [T_out] -> Bus Creator2/1  "T_out"
  [Mdot] -> Bus Creator2/2  "Mdot"
  Pipe_P_to_M/1(x_dot) -> Integrate1/1
  Integrate1/1 -> Pipe_P_to_M/1(x), [T_out]
  [T_in] -> Pipe_P_to_M/2(T_in)
  [T_out] -> n-D Lookup Table1/2
  [P_out] -> n-D Lookup Table1/1
  n-D Lookup Table1/1 -> Mdot/3(Rho), Pipe_P_to_M/4(Rho)
  [P_in] -> Mdot/1(P_in)
  [P_out] -> Mdot/2(P_out)
  Switch/1 -> [Mdot], Pipe_P_to_M/3(Mdot)
  Mdot/1(Mdot) -> Switch/1
  Constant/1 -> Switch/3
  [On_off] -> Switch/2

== system DAEMOT_Lib/Legacy Components/Static Flow Junction ==
  In1 : Inport
  In2 : Inport  Port=2
  Add : Sum
  Add1 : Sum
  Add2 : Sum
  Bus Creator : BusCreator  Inputs=3
  Constant : Constant  Value=2
  Divide1 : Product  Inputs=**
  Divide2 : Product  Inputs=**
  Divide_last : Product  Inputs=/*
  Divide_last1 : Product  Inputs=/*
  b1 : BusSelector  OutputSignals=mdot_kgps,T_C,P_kPa
  b2 : BusSelector  OutputSignals=mdot_kgps,T_C,P_kPa
  Out1 : Outport  VectorParamsAs1DForOutWhenUnconnected=off
  wires:
  Divide1/1 -> Add1/1
  Add1/1 -> Divide_last/2
  [T_in1] -> Divide1/2
  [m_in1] -> Divide1/1
  Divide_last/1 -> [T_out]
  [m_in1] -> Add/1
  Add/1 -> [m_out]
  [T_out] -> Bus Creator/2  "T_C"
  [m_out] -> Bus Creator/1  "mdot_kgps"
  Bus Creator/1 -> Out1/1
  [m_out] -> Divide_last/1
  [P_out] -> Bus Creator/3  "P_kPa"
  b1/1 -> [m_in1]  "<mdot_kgps>"
  b1/2 -> [T_in1]  "<T_C>"
  In1/1 -> b1/1
  b1/3 -> [P_in1]  "<P_kPa>"
  [P_in1] -> Add2/1
  Add2/1 -> Divide_last1/2
  Divide_last1/1 -> [P_out]
  Constant/1 -> Divide_last1/1
  In2/1 -> b2/1
  b2/1 -> [m_in2]  "<mdot_kgps>"
  b2/2 -> [T_in2]  "<T_C>"
  b2/3 -> [P_in2]  "<P_kPa>"
  [m_in2] -> Add/2
  [P_in2] -> Add2/2
  [m_in2] -> Divide2/1
  [T_in2] -> Divide2/2
  Divide2/1 -> Add1/2

== system DAEMOT_Lib/Legacy Components/Static Flow Split ==
  In1 : Inport
  Add : Sum
  Bus Selector : BusSelector  OutputSignals=mdot_kgps,T_C,P_kPa
  Sink1 : Subsystem
      settings: CopyFcn=rev_comms_sink()  NameChangeFcn=rev_comms_sink()
      mask Display: text(0.25,0.5,'Sink')
  Source1 : Subsystem
      mask init:
      | n_src = gcb;
      | n_src = str2num(n_src(end));
      | 
      | rev_comms_source(n_src);
      mask Display: text(0.25,0.5,'Source')
  Source2 : $bdroot/Support Functions/Source
  Terminator : Terminator
  b1 : BusCreator  Inputs=3
  b2 : BusCreator  Inputs=3
  Out1 : Outport  VectorParamsAs1DForOutWhenUnconnected=off
  Out2 : Outport  Port=2  VectorParamsAs1DForOutWhenUnconnected=off
  wires:
  b1/1 -> Out1/1
  [m_dot1] -> b1/1  "mdot_kgps"
  Bus Selector/2 -> [T_in]  "<T_C>"
  [T_in] -> b1/2  "T_C"
  Bus Selector/1 -> Terminator/1  "<mdot_kgps>"
  Source1/1(Out1) -> [m_dot1], Add/1
  In1/1 -> Bus Selector/1
  Add/1 -> Sink1/1(In1)
  [P_in] -> b1/3  "P_kPa"
  Bus Selector/3 -> [P_in]  "<P_kPa>"
  [m_dot2] -> b2/1  "mdot_kgps"
  [T_in] -> b2/2  "T_C"
  [P_in] -> b2/3  "P_kPa"
  b2/1 -> Out2/1
  Source2/1 -> [m_dot2], Add/2

== system DAEMOT_Lib/Legacy Components/Switch ==
  In : Inport
  u : Inport  Port=2
  Bus Creator1 : BusCreator  Inputs=2
  Bus Selector : BusSelector  OutputSignals=V,I
  Product : Product
  Product1 : Product
  Sink1 : $bdroot/Support Functions/Sink
  Source1 : $bdroot/Support Functions/Source
  Terminator3 : Terminator
  Out : Outport  VectorParamsAs1DForOutWhenUnconnected=off
  wires:
  Product/1 -> Bus Creator1/1  "V"
  Bus Creator1/1 -> Out/1
  In/1 -> Bus Selector/1
  Product1/1 -> Sink1/1, Bus Creator1/2  "I"
  Bus Selector/2 -> Terminator3/1  "<I>"
  Bus Selector/1 -> Product/1  "<V>"
  u/1 -> Product1/1, Product/2
  Source1/1 -> Product1/2  "I"

== system DAEMOT_Lib/Legacy Components/To LabVIEW_Old ==
  " " : Inport
  UDP Send : instrumentlib/UDP Send  Host=localhost  Port=61556  LocalPort=61557  EnablePortSharing=off  ByteOrder=BigEndian  OutputDatagramPacketSize=512  EnableBlockingMode=on  LocalAddress=0.0.0.0
      settings: SourceProductName=Instrument Control Toolbox
  Zero-Order Hold : ZeroOrderHold  Commented=through  SampleTime=0.1
  wires:
  " "/1 -> Zero-Order Hold/1
  Zero-Order Hold/1 -> UDP Send/1

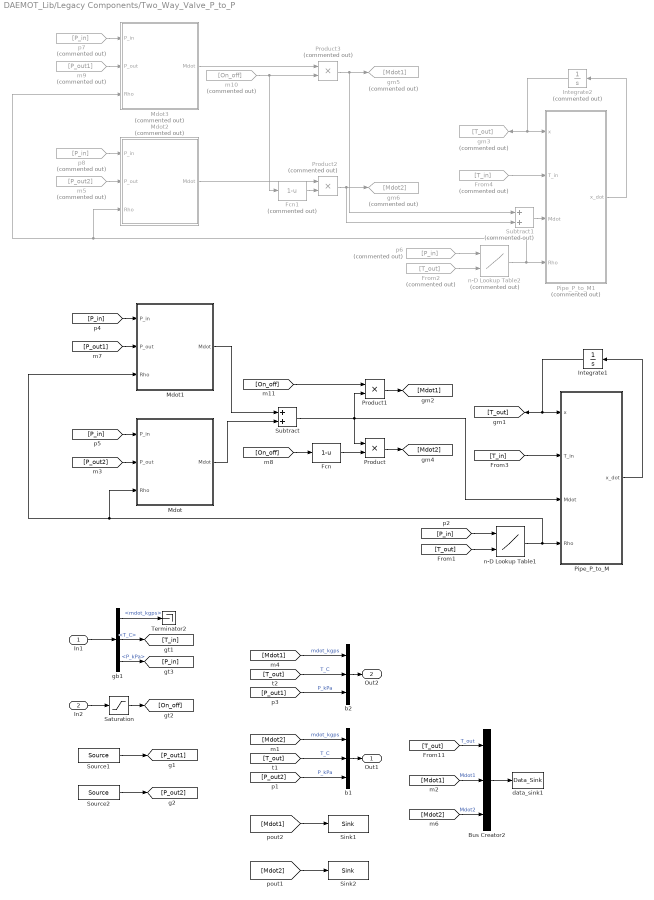
== system DAEMOT_Lib/Legacy Components/Two_Way_Valve_P_to_P ==
  In1 : Inport
  In2 : Inport  Port=2
  Bus Creator2 : BusCreator  Inputs=3
  Fcn : Fcn  Expr=1-u
  Fcn1 : Fcn  Commented=on  Expr=1-u
  From2 : From  Commented=on  GotoTag=T_out
      settings: CloseFcn=tagdialog Close
  From4 : From  Commented=on  GotoTag=T_in
      settings: CloseFcn=tagdialog Close
  Integrate1 : Integrator  InitialCondition=T_init
  Integrate2 : Integrator  Commented=on  InitialCondition=T_init
  Mdot : MATLAB Function  TreatAsAtomicUnit=on
  Mdot1 : MATLAB Function  TreatAsAtomicUnit=on
  Mdot2 : MATLAB Function  Commented=on  TreatAsAtomicUnit=on
  Mdot3 : MATLAB Function  Commented=on  TreatAsAtomicUnit=on
  Pipe_P_to_M : MATLAB Function  TreatAsAtomicUnit=on
  Pipe_P_to_M1 : MATLAB Function  Commented=on  TreatAsAtomicUnit=on
  Product : Product
  Product1 : Product
  Product2 : Product  Commented=on
  Product3 : Product  Commented=on
  Saturation : Saturate  UpperLimit=1  LowerLimit=0
  Sink1 : $bdroot/Support Functions/Sink
  Sink2 : $bdroot/Support Functions/Sink
  Source1 : $bdroot/Support Functions/Source
  Source2 : $bdroot/Support Functions/Source
  Subtract : Sum
  Subtract1 : Sum  Commented=on
  Terminator2 : Terminator
  b1 : BusCreator  Inputs=3
  b2 : BusCreator  Inputs=3
  data_sink1 : $bdroot/Support Functions/Data_Sink
  gb1 : BusSelector  OutputSignals=mdot_kgps,T_C,P_kPa
  gm3 : Goto  Commented=on  GotoTag=T_out
  gm5 : Goto  Commented=on  GotoTag=Mdot1
  gm6 : Goto  Commented=on  GotoTag=Mdot2
  m10 : From  Commented=on  GotoTag=On_off
      settings: CloseFcn=tagdialog Close
  m5 : From  Commented=on  GotoTag=P_out2
      settings: CloseFcn=tagdialog Close
  m9 : From  Commented=on  GotoTag=P_out1
      settings: CloseFcn=tagdialog Close
  n-D Lookup Table1 : Lookup_n-D  BreakpointsForDimension1=Fluid.P  BreakpointsForDimension2=Fluid.T  BreakpointsForDimension3=[5, 7]  Table=Fluid.Rho_pt  ExtrapMethod=Clip  UseLastTableValue=on  RndMeth=Simplest  InputSameDT=on
  n-D Lookup Table2 : Lookup_n-D  Commented=on  BreakpointsForDimension1=Fluid.P  BreakpointsForDimension2=Fluid.T  BreakpointsForDimension3=[5, 7]  Table=Fluid.Rho_pt  ExtrapMethod=Clip  UseLastTableValue=on  RndMeth=Simplest  InputSameDT=on
  p6 : From  Commented=on  GotoTag=P_in
      settings: CloseFcn=tagdialog Close
  p7 : From  Commented=on  GotoTag=P_in
      settings: CloseFcn=tagdialog Close
  p8 : From  Commented=on  GotoTag=P_in
      settings: CloseFcn=tagdialog Close
  Out1 : Outport  VectorParamsAs1DForOutWhenUnconnected=off
  Out2 : Outport  Port=2  VectorParamsAs1DForOutWhenUnconnected=off
  wires:
  Saturation/1 -> [On_off]
  [On_off] -> Fcn/1
  Product/1 -> [Mdot2]
  [P_out2] -> Mdot/2(P_out)
  [P_in] -> Mdot/1(P_in)
  n-D Lookup Table1/1 -> Pipe_P_to_M/4(Rho), Mdot/3(Rho), Mdot1/3(Rho)
  [P_in] -> n-D Lookup Table1/1
  [T_out] -> n-D Lookup Table1/2
  [T_in] -> Pipe_P_to_M/2(T_in)
  Integrate1/1 -> [T_out], Pipe_P_to_M/1(x)
  Pipe_P_to_M/1(x_dot) -> Integrate1/1
  [Mdot1] -> Bus Creator2/2  "Mdot1"
  [T_out] -> Bus Creator2/1  "T_out"
  Bus Creator2/1 -> data_sink1/1
  In2/1 -> Saturation/1
  Source1/1 -> [P_out1]
  [Mdot1] -> Sink1/1
  gb1/3 -> [P_in]  "<P_kPa>"
  [P_out2] -> b1/3  "P_kPa"
  In1/1 -> gb1/1
  gb1/1 -> Terminator2/1  "<mdot_kgps>"
  [T_out] -> b1/2  "T_C"
  gb1/2 -> [T_in]  "<T_C>"
  [Mdot2] -> b1/1  "mdot_kgps"
  b1/1 -> Out1/1
  Source2/1 -> [P_out2]
  [P_out1] -> b2/3  "P_kPa"
  b2/1 -> Out2/1
  [Mdot1] -> b2/1  "mdot_kgps"
  [T_out] -> b2/2  "T_C"
  [Mdot2] -> Sink2/1
  [Mdot2] -> Bus Creator2/3  "Mdot2"
  [P_out1] -> Mdot1/2(P_out)
  [P_in] -> Mdot1/1(P_in)
  Fcn/1 -> Product/2
  Subtract/1 -> Product/1, Product1/2, Pipe_P_to_M/3(Mdot)
  Subtract1/1 -> Pipe_P_to_M1/3(Mdot)
  Fcn1/1 -> Product2/2
  p7/1 -> Mdot3/1(P_in)
  p8/1 -> Mdot2/1(P_in)
  Product2/1 -> Subtract1/2, gm6/1
  m10/1 -> Fcn1/1, Product3/2
  Product3/1 -> Subtract1/1, gm5/1
  m9/1 -> Mdot3/2(P_out)
  Pipe_P_to_M1/1(x_dot) -> Integrate2/1
  m5/1 -> Mdot2/2(P_out)
  From4/1 -> Pipe_P_to_M1/2(T_in)
  p6/1 -> n-D Lookup Table2/1
  From2/1 -> n-D Lookup Table2/2
  Integrate2/1 -> gm3/1, Pipe_P_to_M1/1(x)
  Mdot3/1(Mdot) -> Product3/1
  n-D Lookup Table2/1 -> Pipe_P_to_M1/4(Rho), Mdot2/3(Rho), Mdot3/3(Rho)
  Mdot2/1(Mdot) -> Product2/1
  Mdot1/1(Mdot) -> Subtract/1
  Mdot/1(Mdot) -> Subtract/2
  Product1/1 -> [Mdot1]
  [On_off] -> Product1/1

== system DAEMOT_Lib/Legacy Components/UDP_Controller_SR_old ==
  Controller Input : Inport
  Abs5 : Abs
  Add10 : Sum  Inputs=+-
  Data Type Conversion1 : DataTypeConversion  OutDataTypeStr=double
  From Controller : Subsystem  TreatAsAtomicUnit=on  SystemSampleTime=0.1
  Memory9 : Memory
  Pulse Generator3 : DiscretePulseGenerator  PulseType=Time based  Period=2*update_rate  PulseWidth=50
  Reshape11 : Reshape  OutputDimensionality=Column vector (2-D)
  Sample and Hold : dspsigops/Sample and Hold  trig=Rising edge  initCond=[25.0755482718706,25.0084399359018,25.6133772539970,25.4410284497342,29.2442868126468,24.9995976157054,24.9874035114768,25.4172601295911,25.4038082025570,24.5432998363409,24.7926180342518,24.9028031818592,25.3947015515277,21.9001008266555,21.4191392609994,20.7355591682729,27.8254337424228,24.9227130079907,24.9363515215635,24.8383443019113,24.8698135117088,0.0905255000000000,0.0821940000000000,0.0821940000000000,0,0.137750000000000,0,0.133000000000000,0.134330000000000,0.368125000000000,750,1474.74474028738,25.0553587847645,24.1800648995495,25.3765217260768,25.2885154244095,29.1722865063372,24.0423464609328,23.8449648330486,25.2762757897608,25.2693362310078,22.0888693156576,20.2834883036944,22.3112496474473,24.4829148528305,19.3508626602991,18.6358292867017,17.6173119070624,27.4692798482161,22.6958283453281,22.9629155807725,19.9062771677613,19.6371229254019,25.2355198538971,23.7575725818742,25.6415059744396,25.5899511397452,30.5464153809801,23.5316055587895,23.2098430736181,25.5827275478348,25.5786256324004,20.2671542540310,19.3568501285682,21.4320064115085,23.9173940613866,19.1274076640933,18.4601540221904,17.5097269642686,27.7153254783548,21.8330057261020,22.1131345657598,19.1644017927509,19.0266745049826,25.1151325981121,26.5903473435623,26.0720087684405,25.7378944825845,29.3848893089061,26.8269477734531,27.1672819527981,25.6919928473087,25.6660355466743,27.7944506617566,33.1185045060487,29.7490469824721,27.1384043864179,24.7271320068734,24.4095188178017,23.9617956469169,28.5146883810846,29.1031947447896,28.6533340007561,34.1885659799502,34.9443972575702,25.7668326288005,27.6821718532310,27.6791419425943,27.3241939238173,31.7061243242922,27.9858952214287,28.4215459799927,27.2748222270336,27.2468295681489,29.5999705340445,34.0303633853872,30.9731692008361,30.1850615482580,25.7899612526886,25.2005980000482,24.3669756581712,36.7309137171709,30.3806411294097,29.9664250175689,34.9174715519283,35.5434395349607,0.975388859860216]'  latchinput=off
  Scope3 : Scope
  To Controller : Subsystem  TreatAsAtomicUnit=on  SystemSampleTime=update_rate
  Controller Output : Outport  VectorParamsAs1DForOutWhenUnconnected=off
  wires:
  Controller Input/1 -> Reshape11/1
  From Controller/1(Out1) -> Sample and Hold/1
  Abs5/1 -> Data Type Conversion1/1, Scope3/1
  Sample and Hold/1 -> Controller Output/1
  Data Type Conversion1/1 -> Sample and Hold/Trigger
  Pulse Generator3/1 -> Memory9/1, Add10/1
  Memory9/1 -> Add10/2
  Add10/1 -> Abs5/1
  Reshape11/1 -> To Controller/1(" ")

== system DAEMOT_Lib/Legacy Components/UDP_Controller_old ==
  Controller : MATLABFcn  MATLABFcn=Ctrl_Fcn(u)
  From Controller : Subsystem  TreatAsAtomicUnit=on  SystemSampleTime=1
  Reshape1 : Reshape  OutputDimensionality=Column vector (2-D)
  To Controller : Subsystem  mask{n_meas=in_size}
      mask prompts: n_meas "Number of measurements from LabView"
      mask init:
      | h = gcbh;
      | param = get(h);
      | blk = [param.Path, '/', param.Name,'/UDP Receive'];
      | h = get_param(blk,'handle');
      | 
      | set_param(h,'DataSize',['[',num2str(n_meas),' 1]'])
      mask Display:
      | if n_meas > 1
      |     port_label('output',1,['Mux - ',num2str(n_meas),' signals'])
      | else
      |     port_label('output',1,['Mux - ',num2str(n_meas),' signal'])
      | end
  wires:
  To Controller/1(Out) -> Reshape1/1
  Controller/1 -> From Controller/1(" ")
  Reshape1/1 -> Controller/1

== system DAEMOT_Lib/Legacy Components/Upper to Lower Edge Preview_old ==
  Trajectory : Inport
  Digital Clock : DigitalClock  SampleTime=dt_u
  Mission Preview1 : Subsystem  TreatAsAtomicUnit=on  SystemSampleTime=dt_l
  Reference : Outport  VectorParamsAs1DForOutWhenUnconnected=off
  wires:
  Mission Preview1/1(References) -> Reference/1
  Trajectory/1 -> Mission Preview1/1(Trajectory)
  Digital Clock/1 -> Mission Preview1/2(Time)

== system DAEMOT_Lib/Legacy Components/Wall ==
  In3 : Inport
  Bus Creator2 : BusCreator  Inputs=1
  Integrate : Integrator  InitialCondition=Tw_init
  Mux_In_2 : Mux  Inputs=1
  Q_BUS1 : BusSelector  OutputSignals=Q_kW
  Wall : MATLAB Function  TreatAsAtomicUnit=on
  b1 : BusCreator  Inputs=1
  data_sink1 : $bdroot/Support Functions/Data_Sink
  s1 : $bdroot/Support Functions/Source
  o1 : Outport  VectorParamsAs1DForOutWhenUnconnected=off
  wires:
  Mux_In_2/1 -> Wall/2(Q_fluid)
  [Q_fluid1] -> Mux_In_2/1
  In3/1 -> Q_BUS1/1
  Q_BUS1/1 -> Wall/1(Q_load)  "<Q_kW>"
  [T_wall] -> Bus Creator2/1  "T_wall"
  Bus Creator2/1 -> data_sink1/1
  Wall/1(x_dot) -> Integrate/1
  Integrate/1 -> [T_wall]
  s1/1 -> [Q_fluid1]
  [T_wall] -> b1/1  "T_wall"
  b1/1 -> o1/1

== system DAEMOT_Lib/Support Functions/Data Manager ==
  Data : Outport  VectorParamsAs1DForOutWhenUnconnected=off

== system DAEMOT_Lib/Support Functions/Data_Sink ==
  " " : Inport
  tag scope: gdata_SupportFunctionsData_Sink=global
  wires:
  " "/1 -> [gdata_SupportFunctionsData_Sink]

== system DAEMOT_Lib/Support Functions/Generic Graph Model ==
  Inputs : Inport
  Source Vertex : Inport  Port=2
  Source Edge : Inport  Port=3
  Variant Subsystem : Subsystem  VariantControlMode=Label  Variant=on  LabelModeActiveChoice=DAE_Graph
  States : Outport
  Power Flows : Outport  Port=2
  wires:
  Source Vertex/1 -> Variant Subsystem/2(Source Vertex)
  Inputs/1 -> Variant Subsystem/1(Inputs)
  Source Edge/1 -> Variant Subsystem/3(Source Edge)
  Variant Subsystem/1(States) -> States/1
  Variant Subsystem/2(Power Flows) -> Power Flows/1

== system DAEMOT_Lib/Support Functions/Generic Sink ==
  In1 : Inport
  Sink1 : Subsystem  LoadFcn=rev_comms_sink();  InitFcn=rev_comms_sink();  mask(Sink){}
      mask help: Used for sending data to the upstream component.
      settings: CopyFcn=rev_comms_sink();  NameChangeFcn=rev_comms_sink();
      mask Display: text(0.25,0.5,'Sink')
  Terminator : Terminator
  val : Constant  Value=value
  wires:
  In1/1 -> Terminator/1
  val/1 -> Sink1/1(In1)

== system DAEMOT_Lib/Support Functions/Generic Source ==
  Constant : Constant  Value=0
  Source1 : Subsystem  mask(Source){}
      mask help: Used for receiving data from the downstream component.
      mask init:
      | n_src = gcb;
      | n_src = str2num(n_src(end));
      | try
      |     rev_comms_source(n_src);
      | catch
      | 
      | end
      mask Display: text(0.25,0.5,'Source')
  Terminator : Terminator
  b1 : BusCreator  Inputs=2
  val : Constant  Value=value
  Out1 : Outport  VectorParamsAs1DForOutWhenUnconnected=off
  wires:
  Constant/1 -> b1/1  "current"
  Source1/1(Out1) -> Terminator/1
  b1/1 -> Out1/1
  val/1 -> b1/2  "voltage"

== system DAEMOT_Lib/Support Functions/Mission Preview ==
  1-D Lookup Table : Lookup_n-D  NumberOfTableDimensions=1  BreakpointsForDimension1=timeseries.time  Table=timeseries.data  InterpMethod=Flat  ExtrapMethod=Clip  InternalRulePriority=Speed  RndMeth=Simplest  InputSameDT=on
  Bias : Bias  Bias=+DT*linspace(0,(hor-1),hor)
  Digital Clock : DigitalClock  SampleTime=DT
  Display : Display
  Gain : Gain
  Reshape : Reshape  OutputDimensionality=Row vector (2-D)
  Preview : Outport  VectorParamsAs1DForOutWhenUnconnected=off
  wires:
  1-D Lookup Table/1 -> Reshape/1
  Digital Clock/1 -> Gain/1
  Bias/1 -> 1-D Lookup Table/1
  Reshape/1 -> Display/1, Preview/1
  Gain/1 -> Bias/1
